simulink model "SIM_PEM_single"  (R2020b)
settings: Solver=ode23tb  StartTime=0.0  StopTime=20000  RelTol=1e-4  AbsTol=1e-3  EnableMultiTasking=on
undefined symbols (not defined in the file or in its folder): FC, FuelCellLoadFcn, gcbh, sps_rtmsupport
libraries: powerlib x18, simulink x13, electricdrivelib x10, dspswit3 x1, spsFuelCellModel x1
settings Model: Creator=MathWorks  LastModifiedBy=janluca
settings SolverCC: AutoScaleAbsTol=off
settings DataIOCC: LimitDataPoints=on  SaveFormat=Array  SignalLoggingSaveFormat=ModelDataLogs  ReturnWorkspaceOutputs=off
settings OptimizationCC: ExpressionDepthLimit=2147483647  InitFltsAndDblsToZero=on  EfficientMapNaN2IntZero=off  LifeSpan=inf
settings DebuggingCC: SaveWithParameterizedLinksMsg=none  UnderspecifiedInitializationDetection=Classic  MergeDetectMultiDrivingBlocksExec=none  FcnCallInpInsideContextMsg=warning  AllowSymbolicDim=off  StateNameClashWarn=warning  SFUnexpectedBacktrackingDiag=warning  SFNoUnconditionalDefaultTransitionDiag=warning  SFExecutionAtInitializationDiag=none  ArithmeticOperatorsInVariantConditions=warning
settings HardwareCC: ProdBitPerPointer=32  ProdBitPerSizeT=32  ProdBitPerPtrDiffT=32  ProdLargestAtomicFloat=None  ProdIntDivRoundTo=Undefined  ProdEndianess=Unspecified  ProdWordSize=32  ProdHWDeviceType=32-bit Generic
settings ModelReferenceCC: PropagateSignalLabelsOutOfModel=off
settings SFSimCC: SimUseLocalCustomCode=off  CustomCodeUndefinedFunction=UseInterfaceOnly
settings RTWCC: RTWUseLocalCustomCode=off
settings CodeAppCC: StateflowObjectComments=on
settings GRTTargetCC: TargetFcnLib=ansi_tfl_tmw.mat  TargetLangStandard=C89/C90 (ANSI)  CombineOutputUpdateFcns=off  GRTInterface=on
settings ConfigComp: CovMetricSettings=dw  CovSaveCumulativeToWorkspaceVar=on  CovSaveSingleToWorkspaceVar=on  CovExternalEMLEnable=off  CovSFcnEnable=off
settings SimscapeCC: SimscapeNormalizeSystem=off

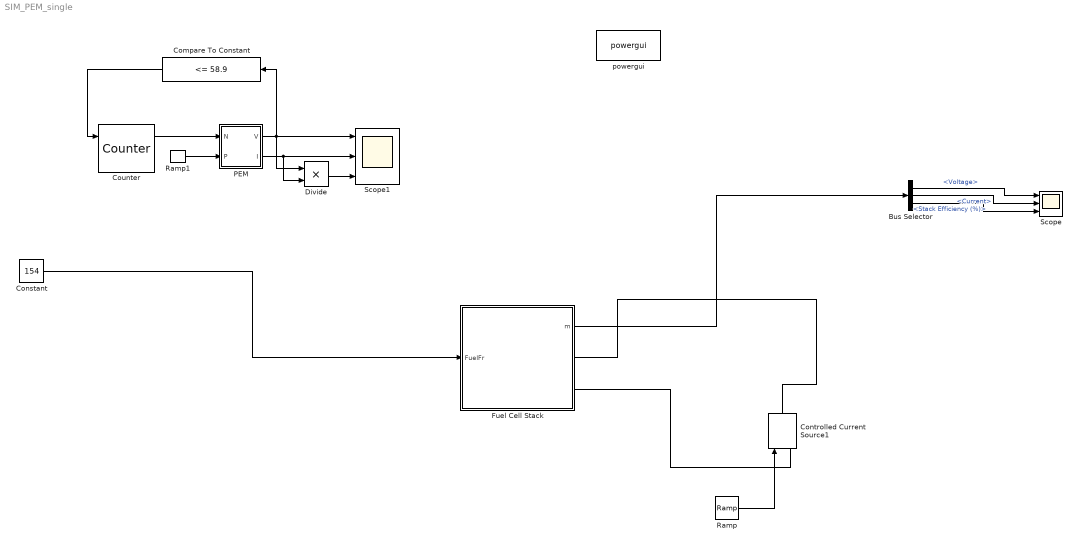
== system SIM_PEM_single ==
  Bus Selector : BusSelector  OutputSignals=Voltage,Current,Stack Efficiency (%)
  Compare To Constant : simulink/Logic and Bit Operations/Compare To Constant  relop=<=  const=58.9  OutDataTypeStr=boolean
  Constant : Constant  Value=154
  Controlled Current Source1 : powerlib/Electrical Sources/Controlled Current Source  Initialize=on  Source_Type=AC  Amplitude=0  Phase=0  Frequency=0  Measurements=None
  Counter : dspswit3/Counter  Direction=Up  CountEvent=Rising edge  CounterSize=User defined  MaxCount=255  InitialCount=1  Output=Count and Hit  HitValue=32  ResetInput=on  SamplesPerFrame=1  Ts=1  CntDtype=double  HitDtype=Logical
  Divide : Product  Inputs=**
  Fuel Cell Stack : Subsystem  AncestorBlock=electricdrivelib/Extra Sources/Fuel Cell Stack  DialogController=POWERSYS.PowerSysDialog  LoadFcn=sps_rtmsupport('LoadFcn',gcbh);FuelCellLoadFcn(gcb)  StartFcn=sps_rtmsupport('StartFcn',gcbh);  StopFcn=sps_rtmsupport('StopFcn',gcbh);  mask(Fuel Cell Stack){PresetModel=No (User-Defined), FcType=Proton Exchange Membrane (PEM), Detailed=Detailed, Eoc=[93.2,88], NomVI=[160,65.5], EndVI=[230,58.9], Nc=96, n=54, TOp=65, AirFr=509, SuppPress=[1.225,1], Comp=[99.95,21,1], SignX=off, SignY=off, FlowRateH2=on, FlowRateAir=off, SystemTemp=off, SystemPH2=off, SystemPAir=off, FCDyn=off, FC_tau=0, Peak_O2=80, V_Under=10}
      mask prompts: PresetModel "Preset model:"; FcType "Fuel Cell type:"; Detailed "Model detail Level:"; Eoc "Voltage at 0A and 1A [V_0(V), V_1(V)]"; NomVI "Nominal operating point [Inom(A), Vnom(V)]"; EndVI "Maximum operating point [Iend(A), Vend(V)]"; Nc "Number of cells"; n "Nominal stack efficiency (%)"; TOp "Operating temperature (Celsius)"; AirFr "Nominal Air flow rate (lpm)"; SuppPress "Nominal supply pressure [Fuel (bar), Air (bar)]"; Comp "Nominal composition (%) [H2 O2 H2O(Air)]"; SignX "Fuel  composition [x_H2(%)]"; SignY "Oxidant composition [y_O2(%)]"; FlowRateH2 "Fuel flow rate [FuelFr(lpm)]"; FlowRateAir "Air flow rate [AirFr(lpm)]"; SystemTemp "System Temperature [T(Kelvin)]"; SystemPH2 "Fuel supply pressure [Pfuel(bar)]"; SystemPAir "Air supply pressure [PAir(bar)]"; FCDyn "Specify Fuel Cell Dynamics?"; FC_tau "Fuel Cell response time (sec)"; Peak_O2 "Peak O2 utilization (%)"; V_Under "Voltage undershoot (V) @ peak O2 utilization"
      mask help:
      | Implements a generic hydrogen fuel cell model which allows the simulation for the following types of cells:
      | - Proton Exchange Membrane Fuel Cell (PEMFC)
      | - Solid Oxide Fuel Cell (SOFC)
      | - Alkaline Fuel Cell (AFC)
      mask init:
      | block = gcb;
      | %% DO NOT CHANGE THIS ORDER
      | FuelCellCback(block,'Inputs')
      | [FC, WantBlockChoice, Ts] = FuelCellInit(block,Eoc,NomVI,EndVI,Nc,n,TOp,AirFr,SuppPress,Comp,FlowRateH2,FlowRateAir);
      | powericon('SetInternalModels','set',block,WantBlockChoice);
      settings: CopyFcn=sps_rtmsupport('CopyFcn',gcbh);  DeleteFcn=sps_rtmsupport('DeleteFcn',gcbh);  UndoDeleteFcn=sps_rtmsupport('UndoDeleteFcn',gcbh);  ModelCloseFcn=sps_rtmsupport('ModelCloseFcn',gcbh);  PreSaveFcn=sps_rtmsupport('PreSaveFcn',gcbh);  PostSaveFcn=sps_rtmsupport('PostSaveFcn',gcbh);  NameChangeFcn=sps_rtmsupport('NameChangeFcn',gcbh);  PreCopyFcn=sps_rtmsupport('PreCopyFcn',gcbh);  OpenFcn=sps_rtmsupport('OpenFcn',gcbh, [1 2 3 13 14 15 16 17 18 19 20]);  CloseFcn=sps_rtmsupport('CloseFcn',gcbh);  PreDeleteFcn=sps_rtmsupport('PreDeleteFcn',gcbh);
      mask Help: helpview(psbhelp)
      mask TypeOptions PresetModel: No (User-Defined) | PEMFC - 1.26 kW - 24 Vdc | PEMFC - 6 kW - 45 Vdc | PEMFC - 50 kW - 625 Vdc | AFC - 2.4 kW - 48 Vdc | SOFC - 3 kW - 100 Vdc | SOFC - 25 kW - 630 Vdc
      mask Callback PresetModel: FuelCellCback(gcb,'Preset')
      mask TypeOptions Detailed: Simplified | Detailed
      mask Callback Detailed: FuelCellCback(gcb,'Visibilities')
      mask Callback FlowRateAir: FuelCellCback(gcb,'Visibilities')
      mask Callback FCDyn: FuelCellCback(gcb,'Visibilities')
      mask DialogControl ParameterTabVar0 Prompt: Parameters
      mask DialogControl plot_graph Prompt: Plot V_I characteristic
      mask DialogControl plot_graph Callback: FuelCellCback(gcb,'PlotGraph');
      mask DialogControl ViewParam Prompt: View Cell parameters
      mask DialogControl ViewParam Callback: FuelCellCback(gcb,'ViewParam');
      mask DialogControl ParameterTabVar01 Prompt: Signal variation
      mask DialogControl ParameterTabVar012 Prompt: Fuel Cell Dynamics
      mask Display: image(imread('power_fuelcell.png'));
  PEM : Subsystem
  Ramp : simulink/Sources/Ramp  slope=-0.1  start=0  InitialOutput=0
  Ramp1 : simulink/Sources/Ramp  slope=-0.1  start=0  InitialOutput=0
  Scope : Scope  NumInputPorts=3
  Scope1 : Scope  NumInputPorts=3
  powergui : powerlib/powergui  Priority=1  SimulationMode=Continuous  SampleTime=50e-6  frequency=60  Iterations=50  frequencyindice=0  Pbase=100e6  ErrMax=1e-4  UnitsV=kV  UnitsW=MW  buscounter=0  FunctionMessages=off  echomessages=off  EnableUseOfTLC=off  CurrentSourceSwitches=off  DisableSnubberDevices=off  DisableRonSwitches=off  DisableVfSwitches=off  DisplayEquations=off  AutomaticDiscreteSolvers=off  SolverType=Tustin/Backward Euler (TBE)  Interpol=off  ExternalGateDelay=off  methode=off  Ts=100  x0status=blocks  SPID=on  SwTol=0  HookPort=off  NonlinearTolerance=1e-4  nMaxIteration=100  ContinueOnMaxIteration=off  RestoreLinks=warning  ResistiveCurrentMeasurement=off  Frange=[0:2:500]  Ylog=off  Xlog=on  ShowGrid=off  save=off  variable=ZData  structure=0  ZoomFFT=off  StartTime=0.0  cycles=1  DisplayStyle=1  fundamental=60  FreqAxis=off  MaxFrequency=1000  frequencyindicesteady=1  RmsSteady=1  display=off
  wires:
  Ramp/1 -> Controlled Current Source1/1
  Fuel Cell Stack/1(m) -> Bus Selector/1
  Bus Selector/1 -> Scope/1  "<Voltage>"
  Bus Selector/2 -> Scope/2  "<Current>"
  Bus Selector/3 -> Scope/3  "<Stack Efficiency (%)>"
  Constant/1 -> Fuel Cell Stack/1(FuelFr)
  Counter/1 -> PEM/1(N)
  Ramp1/1 -> PEM/2(P)
  PEM/1(V) -> Divide/1, Compare To Constant/1, Scope1/1
  Compare To Constant/1 -> Counter/1
  Divide/1 -> Scope1/3
  PEM/2(I) -> Divide/2, Scope1/2
  connections:
  Fuel Cell Stack/RConn2 -- Controlled Current Source1/LConn1
  Controlled Current Source1/RConn1 -- Fuel Cell Stack/RConn1

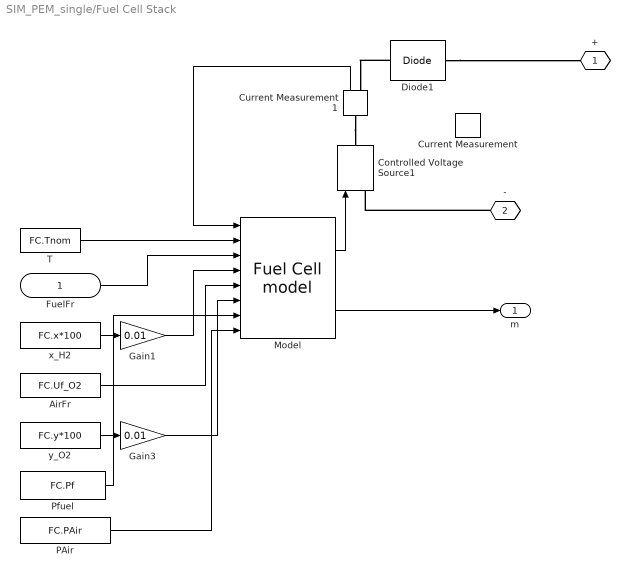
== system SIM_PEM_single/Fuel Cell Stack ==
  FuelFr : Inport
  AirFr : Constant  Value=FC.Uf_O2
  Controlled Voltage Source1 : powerlib/Electrical Sources/Controlled Voltage Source  Initialize=on  Source_Type=AC  Amplitude=0  Phase=0  Frequency=0  Measurements=None
  Current Measurement : powerlib/Measurements/Current Measurement  PhasorSimulation=off  OutputType=Complex  PSBequivalent=0
  Current Measurement1 : powerlib/Measurements/Current Measurement  PhasorSimulation=off  OutputType=Complex  PSBequivalent=0
  Diode1 : powerlib/Power Electronics/Diode  Ron=FC.Rohm  Lon=0  Vf=0  IC=0  UseSnubber=off  Rs=1e4  Cs=inf  Measurements=off
  Gain1 : Gain  Gain=0.01
  Gain3 : Gain  Gain=0.01
  Model : spsFuelCellModel/Fuel Cell model  SystemSampleTime=-1  LabelModeActiveChoice=Continuous/Detailed  VariantActivationTime=update diagram  Latency=0  AutoFrameSizeCalculation=off
      settings: AttributesFormatString=%<BlockChoice>  SourceProductBaseCode=PS
  PAir : Constant  Value=FC.PAir
  Pfuel : Constant  Value=FC.Pf
  T : Constant  Value=FC.Tnom
  x_H2 : Constant  Value=FC.x*100
  y_O2 : Constant  Value=FC.y*100
  + : PMIOPort  Tag=PMCPort  Side=Right
  - : PMIOPort  Tag=PMCPort  Port=2  Side=Right
  m : Outport  VectorParamsAs1DForOutWhenUnconnected=off
  wires:
  PAir/1 -> Model/8
  Pfuel/1 -> Model/7
  T/1 -> Model/2
  Model/1 -> Controlled Voltage Source1/1
  Current Measurement1/1 -> Model/1
  Model/2 -> m/1
  FuelFr/1 -> Model/3
  x_H2/1 -> Gain1/1
  AirFr/1 -> Model/5
  y_O2/1 -> Gain3/1
  Gain1/1 -> Model/4
  Gain3/1 -> Model/6
  connections:
  Current Measurement1/LConn1 -- Controlled Voltage Source1/RConn1
  Diode1/LConn1 -- Current Measurement1/RConn1
  -/RConn1 -- Controlled Voltage Source1/LConn1
  Diode1/RConn1 -- +/RConn1

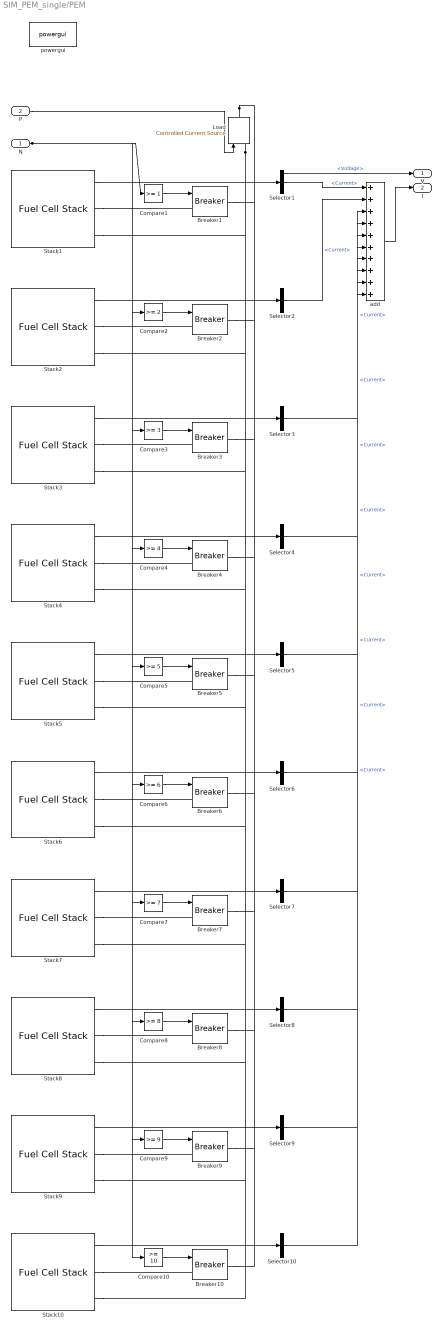
== system SIM_PEM_single/PEM ==
  N : Inport
  P : Inport  Port=2
  Breaker{1..10} (10 alike) : powerlib/Elements/Breaker  InitialState=0  SwitchingTimes="[1/60  5/60]"  External=on  BreakerResistance=0.01  SnubberResistance=1e6  SnubberCapacitance=inf  Measurements=None  MoreParameters=on  NoBreakLoop=off
  Compare1 : simulink/Logic and Bit Operations/Compare To Constant  relop=>=  const=1  OutDataTypeStr=boolean
  Compare10 : simulink/Logic and Bit Operations/Compare To Constant  relop=>=  const=10  OutDataTypeStr=boolean
  Compare2 : simulink/Logic and Bit Operations/Compare To Constant  relop=>=  const=2  OutDataTypeStr=boolean
  Compare3 : simulink/Logic and Bit Operations/Compare To Constant  relop=>=  const=3  OutDataTypeStr=boolean
  Compare4 : simulink/Logic and Bit Operations/Compare To Constant  relop=>=  const=4  OutDataTypeStr=boolean
  Compare5 : simulink/Logic and Bit Operations/Compare To Constant  relop=>=  const=5  OutDataTypeStr=boolean
  Compare6 : simulink/Logic and Bit Operations/Compare To Constant  relop=>=  const=6  OutDataTypeStr=boolean
  Compare7 : simulink/Logic and Bit Operations/Compare To Constant  relop=>=  const=7  OutDataTypeStr=boolean
  Compare8 : simulink/Logic and Bit Operations/Compare To Constant  relop=>=  const=8  OutDataTypeStr=boolean
  Compare9 : simulink/Logic and Bit Operations/Compare To Constant  relop=>=  const=9  OutDataTypeStr=boolean
  Load : powerlib/Electrical Sources/Controlled Current Source  Initialize=on  Source_Type=AC  Amplitude=0  Phase=0  Frequency=0  Measurements=None
  Selector{1..10} (10 alike) : BusSelector  OutputSignals=Voltage,Current,Stack Efficiency (%)
  Stack{1..10} (10 alike) : electricdrivelib/Extra Sources/Fuel Cell Stack  PresetModel=No (User-Defined)  FcType=0  Detailed=Detailed  Eoc=[93.2 88]  NomVI=[160 65.5]  EndVI=[230 58.9]  Nc=96  n=54  TOp=65  AirFr=732  SuppPress=[1.225,1]  Comp=[99.95,21,1]  SignX=off  SignY=off  FlowRateH2=off  FlowRateAir=off  SystemTemp=off  SystemPH2=off  SystemPAir=off  FCDyn=off  FC_tau=1  Peak_O2=80  V_Under=10
      settings: SourceProductBaseCode=PS
  add : Sum  Inputs=++++++++++
  powergui : powerlib/powergui  Priority=1  SimulationMode=Continuous  SampleTime=50e-6  frequency=60  Iterations=50  frequencyindice=60  Pbase=100e6  ErrMax=1e-4  UnitsV=kV  UnitsW=MW  buscounter=0  FunctionMessages=off  echomessages=off  EnableUseOfTLC=off  CurrentSourceSwitches=off  DisableSnubberDevices=off  DisableRonSwitches=off  DisableVfSwitches=off  DisplayEquations=off  AutomaticDiscreteSolvers=off  SolverType=Tustin/Backward Euler (TBE)  Interpol=off  ExternalGateDelay=off  methode=off  Ts=100  x0status=blocks  SPID=on  SwTol=0  HookPort=off  NonlinearTolerance=1e-4  nMaxIteration=100  ContinueOnMaxIteration=off  RestoreLinks=warning  ResistiveCurrentMeasurement=off  Frange=[0:2:500]  Ylog=off  Xlog=on  ShowGrid=off  save=off  variable=ZData  structure=0  ZoomFFT=off  StartTime=0.0  cycles=1  DisplayStyle=1  fundamental=60  FreqAxis=off  MaxFrequency=1000  frequencyindicesteady=1  RmsSteady=1  display=off
  V : Outport
  I : Outport  Port=2
  wires:
  Compare1/1 -> Breaker1/1
  N/1 -> Compare1/1, Compare2/1, Compare3/1, Compare4/1, Compare5/1, Compare6/1, Compare7/1, Compare8/1, Compare9/1, Compare10/1
  Stack1/1 -> Selector1/1
  Selector1/2 -> add/1  "<Current>"
  Selector1/1 -> V/1  "<Voltage>"
  Compare2/1 -> Breaker2/1
  Stack2/1 -> Selector2/1
  Selector2/2 -> add/2  "<Current>"
  Compare3/1 -> Breaker3/1
  Stack3/1 -> Selector3/1
  Selector3/2 -> add/3  "<Current>"
  Compare4/1 -> Breaker4/1
  Stack4/1 -> Selector4/1
  Selector4/2 -> add/4  "<Current>"
  Compare5/1 -> Breaker5/1
  Stack5/1 -> Selector5/1
  Selector5/2 -> add/5  "<Current>"
  Compare6/1 -> Breaker6/1
  Stack6/1 -> Selector6/1
  Selector6/2 -> add/6  "<Current>"
  Compare7/1 -> Breaker7/1
  Stack7/1 -> Selector7/1
  Selector7/2 -> add/7  "<Current>"
  Compare8/1 -> Breaker8/1
  Stack8/1 -> Selector8/1
  Selector8/2 -> add/8  "<Current>"
  Compare9/1 -> Breaker9/1
  Stack9/1 -> Selector9/1
  Selector9/2 -> add/9  "<Current>"
  Compare10/1 -> Breaker10/1
  Stack10/1 -> Selector10/1
  Selector10/2 -> add/10  "<Current>"
  P/1 -> Load/1
  add/1 -> I/1
  connections:
  Stack1/RConn1 -- Breaker1/LConn1
  Breaker1/RConn1 -- Breaker2/RConn1 -- Breaker3/RConn1 -- Breaker4/RConn1 -- Breaker5/RConn1 -- Breaker6/RConn1 -- Breaker7/RConn1 -- Breaker8/RConn1 -- Breaker9/RConn1 -- Load/RConn1 -- Breaker10/RConn1
  Stack1/RConn2 -- Stack2/RConn2 -- Stack3/RConn2 -- Stack4/RConn2 -- Stack5/RConn2 -- Stack6/RConn2 -- Stack7/RConn2 -- Stack8/RConn2 -- Stack9/RConn2 -- Load/LConn1 -- Stack10/RConn2
  Stack2/RConn1 -- Breaker2/LConn1
  Stack3/RConn1 -- Breaker3/LConn1
  Stack4/RConn1 -- Breaker4/LConn1
  Stack5/RConn1 -- Breaker5/LConn1
  Stack6/RConn1 -- Breaker6/LConn1
  Stack7/RConn1 -- Breaker7/LConn1
  Stack8/RConn1 -- Breaker8/LConn1
  Stack9/RConn1 -- Breaker9/LConn1
  Stack10/RConn1 -- Breaker10/LConn1
